simulink model "Q4_sim"  (R2023b)
settings: Solver=VariableStepAuto  StartTime=0.0  StopTime=6  RelTol=1e-3
settings Model: Creator=avikd  LastModifiedBy=avikd

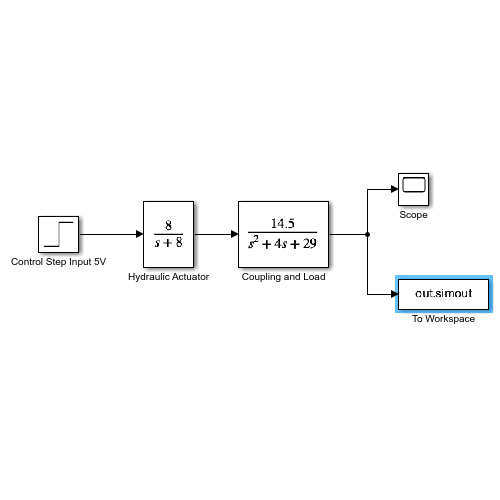
[thumbnail: Simulink's stored preview of the top-level diagram]
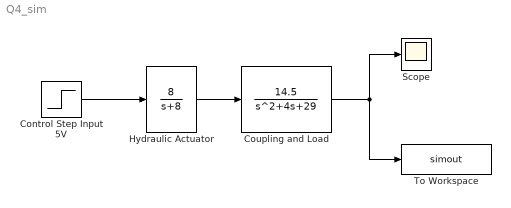
== system Q4_sim ==
  Control Step Input 5V : Step  After=5  SampleTime=0
  Coupling and Load : TransferFcn  Numerator=[14.5]  Denominator=[1 4 29]
  Hydraulic Actuator : TransferFcn  Numerator=[8]  Denominator=[1 8]
  Scope : Scope
  To Workspace : ToWorkspace  VariableName=simout  SaveFormat=Timeseries  SampleTime=0.005
  wires:
  Hydraulic Actuator/1 -> Coupling and Load/1
  Control Step Input 5V/1 -> Hydraulic Actuator/1
  Coupling and Load/1 -> Scope/1, To Workspace/1
